simulink model "testifintegratoriscorrect"  (R2019a)
settings: Solver=FixedStepAuto  StartTime=0.0  StopTime=100  FixedStep=1e-4  RelTol=1e-5
InitFcn:
  | HeightAboveSeaLevel = 400 * rand;
  | Temperature = 288.15 + 30 * (rand - 0.5);
  | Pressure = 	101325 + 6000 * (rand - 0.5);
  | 
  | GustStart = 5 * rand;
  | GustLength = [100 + 50 * (rand - 0.5), 100 + 50 * (rand - 0.5), 100 + 50 * (rand - 0.5)];
  | GuestAmplitude = [ 10 * (rand - 0.5), 10 * (rand - 0.5),  10 * (rand - 0.5)];
  | 
  | ShearSpeed = 20 * rand;
  | ShearDirection = 360 * rand;
  | 
  | HeightAboveSeaLevel = 5.4419142084;
  | Temperature = 288.15;
  | Pressure = 	101325;
  | 
  | GustStart = 2.5;
  | GustLength = [100, 100, 100];
  | GuestAmplitude = [ 2.5, -2.5,  1];
  | 
  | ShearSpeed = 10;
  | ShearDirection = 180;
values from neighbouring files (symbols this model uses):
  D = zeros(size(B))    [RocketOutputFunction.m]    (also in StateSpaceController.m = zeros(13, 3); TimeDelayCompensationElevator.m = [0; 0])
  F = eye(6)    [MEKFAttitudeOnly.m]
  Ki2 = lqr(Ai2, Bi2, Q, R)    [StateSpaceController.m]
  q = x(13:16)    [AdaptiveLQR.m]    (also in MEKF.m = nominal_state(4:7); MEKFAttitudeOnly.m = [1 0 0 0]; MEKF_old.m = nominal_state(4:7); NonlinearStateEstimationForActuatorDelay.m = x(4:7))
  r = sym('r', [3 1])    [StateSpaceController.m]    (also in TimeDelayCompensationElevator.m = [0;0]; Tracker.m = [0; 0; -(rocket_length - Average_cg)])
  s = linspace(0, 100, nums)    [ImpactVelocityFunction.m]    (also in ImpactVelocityNotParallelMatlab.m = 1:5:500; ParallelImpactVelocity.m = .1:.01:500; ParralelRun.m = linspace(5,7, nums); RunImpactVelocityParforCompiled.m = 1:0.1:500)
undefined symbols (not defined in the file or in its folder): deg, e0_0, e1_0, e2_0, e3_0, Earth, Light, magnitude, MIL, rad, WGS84
libraries: aerolibutil x10, simulink x9, aerolibconvert2 x7, sharedtransform x7, shared6dof x7, aerolibwind2 x3, sharedutil x3, aerolibfltsims x2, aerolibasang x2, shared6dofsys x2, aerolibatmos2 x1, aerolibbdyn x1
(part 2 of 2)

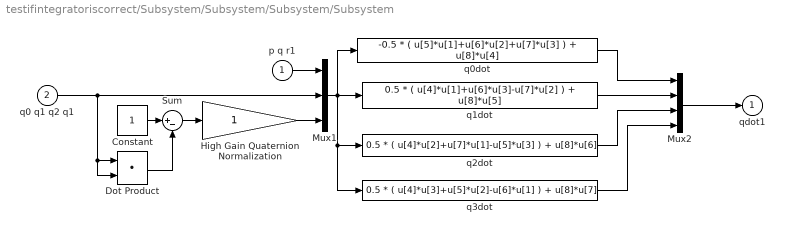
== system testifintegratoriscorrect/Subsystem/Subsystem/Subsystem/Subsystem ==
  p q r1 : Inport
  q0 q1 q2 q1 : Inport  Port=2
  Constant : Constant
  Dot Product : DotProduct  OutDataTypeStr=Inherit: Inherit via internal rule
  High Gain Quaternion Normalization : Gain  SaturateOnIntegerOverflow=on  OutDataTypeStr=Inherit: Same as input  ParamDataTypeStr=Inherit: Same as input
  Mux1 : Mux  Inputs=[3 4 1]
  Mux2 : Mux
  Sum : Sum  Inputs=|+-  SaturateOnIntegerOverflow=on  InputSameDT=on  OutDataTypeStr=Inherit: Same as first input
  q0dot : Fcn  Expr=-0.5 * ( u[5]*u[1]+u[6]*u[2]+u[7]*u[3] ) + u[8]*u[4]
  q1dot : Fcn  Expr=0.5 * ( u[4]*u[1]+u[6]*u[3]-u[7]*u[2] ) + u[8]*u[5]
  q2dot : Fcn  Expr=0.5 * ( u[4]*u[2]+u[7]*u[1]-u[5]*u[3] ) + u[8]*u[6]
  q3dot : Fcn  Expr=0.5 * ( u[4]*u[3]+u[5]*u[2]-u[6]*u[1] ) + u[8]*u[7]
  qdot1 : Outport  InitialOutput=0
  wires:
  Constant/1 -> Sum/1
  Dot Product/1 -> Sum/2
  Mux1/1 -> q2dot/1, q3dot/1, q0dot/1, q1dot/1
  q0 q1 q2 q1/1 -> Dot Product/1, Dot Product/2, Mux1/2
  Sum/1 -> High Gain Quaternion Normalization/1
  Mux2/1 -> qdot1/1
  q0dot/1 -> Mux2/1
  q3dot/1 -> Mux2/4
  q1dot/1 -> Mux2/2
  q2dot/1 -> Mux2/3
  High Gain Quaternion Normalization/1 -> Mux1/3
  p q r1/1 -> Mux1/1

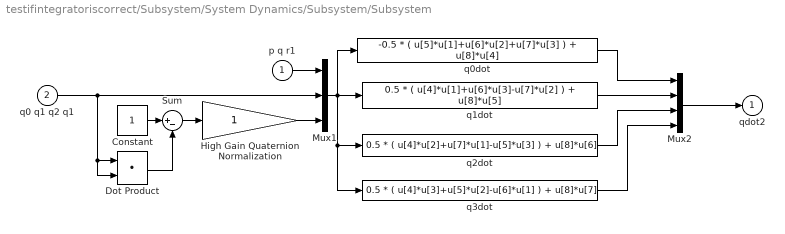
== system testifintegratoriscorrect/Subsystem/System Dynamics/Subsystem/Subsystem ==
  p q r1 : Inport
  q0 q1 q2 q1 : Inport  Port=2
  Constant : Constant
  Dot Product : DotProduct  OutDataTypeStr=Inherit: Inherit via internal rule
  High Gain Quaternion Normalization : Gain  SaturateOnIntegerOverflow=on  OutDataTypeStr=Inherit: Same as input  ParamDataTypeStr=Inherit: Same as input
  Mux1 : Mux  Inputs=[3 4 1]
  Mux2 : Mux
  Sum : Sum  Inputs=|+-  SaturateOnIntegerOverflow=on  InputSameDT=on  OutDataTypeStr=Inherit: Same as first input
  q0dot : Fcn  Expr=-0.5 * ( u[5]*u[1]+u[6]*u[2]+u[7]*u[3] ) + u[8]*u[4]
  q1dot : Fcn  Expr=0.5 * ( u[4]*u[1]+u[6]*u[3]-u[7]*u[2] ) + u[8]*u[5]
  q2dot : Fcn  Expr=0.5 * ( u[4]*u[2]+u[7]*u[1]-u[5]*u[3] ) + u[8]*u[6]
  q3dot : Fcn  Expr=0.5 * ( u[4]*u[3]+u[5]*u[2]-u[6]*u[1] ) + u[8]*u[7]
  qdot2 : Outport
  wires:
  q0 q1 q2 q1/1 -> Dot Product/1, Dot Product/2, Mux1/2
  Mux1/1 -> q2dot/1, q3dot/1, q0dot/1, q1dot/1
  Constant/1 -> Sum/1
  High Gain Quaternion Normalization/1 -> Mux1/3
  q1dot/1 -> Mux2/2
  q0dot/1 -> Mux2/1
  Sum/1 -> High Gain Quaternion Normalization/1
  Dot Product/1 -> Sum/2
  q3dot/1 -> Mux2/4
  Mux2/1 -> qdot2/1
  q2dot/1 -> Mux2/3
  p q r1/1 -> Mux1/1

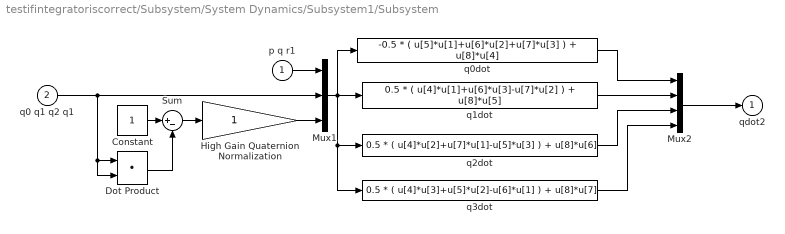
== system testifintegratoriscorrect/Subsystem/System Dynamics/Subsystem1/Subsystem ==
  p q r1 : Inport
  q0 q1 q2 q1 : Inport  Port=2
  Constant : Constant
  Dot Product : DotProduct  OutDataTypeStr=Inherit: Inherit via internal rule
  High Gain Quaternion Normalization : Gain  SaturateOnIntegerOverflow=on  OutDataTypeStr=Inherit: Same as input  ParamDataTypeStr=Inherit: Same as input
  Mux1 : Mux  Inputs=[3 4 1]
  Mux2 : Mux
  Sum : Sum  Inputs=|+-  SaturateOnIntegerOverflow=on  InputSameDT=on  OutDataTypeStr=Inherit: Same as first input
  q0dot : Fcn  Expr=-0.5 * ( u[5]*u[1]+u[6]*u[2]+u[7]*u[3] ) + u[8]*u[4]
  q1dot : Fcn  Expr=0.5 * ( u[4]*u[1]+u[6]*u[3]-u[7]*u[2] ) + u[8]*u[5]
  q2dot : Fcn  Expr=0.5 * ( u[4]*u[2]+u[7]*u[1]-u[5]*u[3] ) + u[8]*u[6]
  q3dot : Fcn  Expr=0.5 * ( u[4]*u[3]+u[5]*u[2]-u[6]*u[1] ) + u[8]*u[7]
  qdot2 : Outport
  wires:
  q0 q1 q2 q1/1 -> Dot Product/1, Dot Product/2, Mux1/2
  Mux1/1 -> q2dot/1, q3dot/1, q0dot/1, q1dot/1
  Constant/1 -> Sum/1
  High Gain Quaternion Normalization/1 -> Mux1/3
  q1dot/1 -> Mux2/2
  q0dot/1 -> Mux2/1
  Sum/1 -> High Gain Quaternion Normalization/1
  Dot Product/1 -> Sum/2
  q3dot/1 -> Mux2/4
  Mux2/1 -> qdot2/1
  q2dot/1 -> Mux2/3
  p q r1/1 -> Mux1/1

== matlab function testifintegratoriscorrect/50Hz delay ==
  settings: updateMethod=DISCRETE
  data: time input; input input; delayed_input output
function delayed_input = Servo(time, input)
    persistent lastupdate
    if isempty(lastupdate)
        lastupdate = [0;0];
    end
    
    servo_frequency = 50; %Hz
    if mod(time, 1/servo_frequency) == 0
        lastupdate = input;
    end    
        
    delayed_input = lastupdate;
end

== matlab function testifintegratoriscorrect/Subsystem/Acceleration Calculator/Subsystem/AngleOfAtack1 ==
  settings: updateMethod=DISCRETE
  data: Airspeed input; AoA output
function AoA = AngleOfAttack(Airspeed)
    AoA = acos(Airspeed(3) / norm(Airspeed));
        
    if norm(Airspeed) <= .01
        AoA = 0;
    end
end

== matlab function testifintegratoriscorrect/Subsystem/Acceleration Calculator/Forces And Moments simple model1 ==
  settings: updateMethod=DISCRETE
  data: Mach input; Airspeed input size=[3 1]; AoA input; Density input; Temperature input; DynamicPressure input; CenterOfMassX input; Thrust input; Forces output; body_angular_velocity input; Xe input; Moments output
function [Forces, Moments]  = forces(Mach, Airspeed, AoA, Density, Temperature, DynamicPressure, CenterOfMassX, Thrust, body_angular_velocity, Xe)
    persistent ThetaRotation
    if isempty(ThetaRotation)
         ThetaRotation = eye(3);
    end
    
    %% Rocket Shape Constants
    Reference_Diameter = 7.62e-2;
    Reference_Radius = Reference_Diameter / 2;
    Reference_Area = Reference_Radius^2 * pi;
    
    NoseCone_Length = 15e-2;
    BodyTube_Length = 80e-2; 
    NoseCone_WetArea = pi * Reference_Radius * NoseCone_Length;          % pi*r*l 
    BodyTube_WetArea = pi * Reference_Radius * 2 * BodyTube_Length;      % pi*d*l
    NoseCone_PlanformArea = Reference_Diameter * NoseCone_Length / 2;
    BodyTube_PlanformArea = Reference_Diameter * BodyTube_Length;
    
    SurfaceRoughness = 20e-6;
    
    sinphi = Reference_Radius / hypot(Reference_Radius, NoseCone_Length);
    BodyTube_CP = 0.55;
    NoseCone_CP = 0.1;
    PitchCenterX = 0;
   
    
    COT_to_COM = .95 - CenterOfMassX; %get actual value and change over time as solid motor burns
    
    %% General Constants
    K = 1.1;
   
    %% Coefficients
    angularrate_local = ThetaRotation \ body_angular_velocity;
    [CN, Cpitch] = CalculatePitchAndNormalCDs(Mach, K, Reference_Diameter, AoA, Airspeed, angularrate_local(2), NoseCone_Length, BodyTube_Length, Reference_Area, CenterOfMassX, PitchCenterX, NoseCone_PlanformArea, BodyTube_PlanformArea, NoseCone_CP, BodyTube_CP);

    Cbase = .12 + .13*Mach^2;
    CFrictionDrag = CalculateFrictionDrag(Temperature, Density, Reference_Radius, Reference_Area, SurfaceRoughness, NoseCone_Length, BodyTube_Length, Airspeed, Mach, NoseCone_WetArea, BodyTube_WetArea);
    Cpressure = PressureDragForce(sinphi);
    
    Cdrag = Cbase + CFrictionDrag + Cpressure;
    Caxial = AxialDragMul(AoA) * Cdrag;

    Cyaw = 0;
    %Croll = 0.003 * (rand - 0.5);
    Croll = 0;
    Cside = 0;
    
     %% Random Noise to pitch and yaw coefficients in the range of +- 5e-4
    %Cpitch = Cpitch + .1 * (rand - 0.5);
    %Cyaw = Cyaw + .1 * (rand - 0.5);
    %Croll = Croll + .00005 * (rand - 0.5);
    %% Forces and Moments
    lengtha = norm(Airspeed(1:2));
    
    sina = Airspeed(2) / lengtha;
    cosa = Airspeed(1) / lengtha;

    ThetaRotation = [cosa, -sina, 0; sina, cosa, 0; 0, 0, 1];
    
    z = DynamicPressure * Reference_Area;
    Thrust_moment = COT_to_COM * [Thrust(2); Thrust(1); 0];
    
    Forces = ThetaRotation * z * -[CN; Cside; Caxial] + Thrust;
    Moments = ThetaRotation * (z * Reference_Diameter * [-Cyaw; Cpitch; Croll]) + Thrust_moment;
    
    if Xe(3) <= 0
        Forces = [0;0;Forces(3)];
        Moments = [0; 0; 0];
    end
    
end

== matlab function testifintegratoriscorrect/Subsystem2/Desired Quaternion ==
  settings: updateMethod=DISCRETE
  data: input_acceleration input; thrust_acceleration input; desired_quaternion output size=[1 4]; ln_quat output
function [desired_quaternion, ln_quat] = func(input_acceleration, thrust_acceleration)

    max_horizontal_acceleration = sin(deg2rad(10)) * thrust_acceleration;
    if norm(input_acceleration) > max_horizontal_acceleration
        input_acceleration = input_acceleration * max_horizontal_acceleration / norm(input_acceleration);
    end
    
    global_thrust = [input_acceleration.', (thrust_acceleration^2 - norm(input_acceleration)^2)^.5];
    
    if norm(global_thrust) == 0
        global_thrust = [0,0,1];
    end
    
    desired_quaternion = quatnormalize([ global_thrust(3) + norm(global_thrust), cross([0;0;1], global_thrust) ]);
%     test = quatnormalize([norm(global_thrust) + global_thrust(3), cross([0 0 1], global_thrust)]);
    
    if norm(desired_quaternion(2:4)) == 0
        ln_quat = [0 0 0];
    else
        ln_quat = desired_quaternion(2:4)/norm(desired_quaternion(2:4)) * desired_quaternion(1);
    end
    
%     desired_quaternion = [cos(pi/8) sin(pi/8) * [1 0 0]];

== matlab function testifintegratoriscorrect/Desired Quaternion ==
  settings: updateMethod=DISCRETE
  data: current_orientation input; desired_quaternion input; current_quaternion output size=[1 4]
function current_quaternion = func(current_orientation, desired_quaternion)
    rotation_b = quatmultiply(quatinv(current_orientation.'), desired_quaternion); %rotation required in body coordinate system

    theta = atan( rotation_b(4) / rotation_b(1) ); %half the roll angle
    roll_b = [cos(theta), 0, 0, sin(theta)]; %extract roll part of quaternion
    noroll_b = quatmultiply(rotation_b, quatinv(roll_b)); %desired rotation in body coordinate system
%     noroll_i = quatmultiply(current_orientation.', quatmultiply(noroll_b, quatinv(current_orientation.')));
    
    current_quaternion = quatnormalize(quatinv( noroll_b )); % then take the inverse to pretend to be at inverse orientation, due to state space being designed like that

    if current_quaternion(1) < 0
        current_quaternion = -current_quaternion;
    end

== matlab function testifintegratoriscorrect/Subsystem/System Dynamics/w to quat ==
  settings: updateMethod=DISCRETE
  data: w input; quaternion output size=[1 4]
function quaternion = func(w)
    quaternion = [cos(norm(w) / 2), sin(norm(w) / 2) * w.' / norm(w)];

== matlab function testifintegratoriscorrect/Subsystem/Desired Quaternion ==
  settings: updateMethod=DISCRETE
  data: current_orientation input; current_quaternion output
function current_quaternion = func(current_orientation)
    current_quaternion = current_orientation;
    
    t = acos(current_quaternion(1));
    if current_quaternion(1) < 0
        current_quaternion(1) = cos(pi - t);
        current_quaternion(2:4) = -current_quaternion(2:4);
    end

== matlab function testifintegratoriscorrect/Subsystem/Acceleration Calculator/Subsystem/Subsystem/DCM ==
  settings: updateMethod=DISCRETE
  data: DCM output
function DCM  = forces
    DCM = [1,0,0;0,1,0;0,0,1];

== matlab function testifintegratoriscorrect/Subsystem/Acceleration Calculator/Subsystem/Subsystem/MATLAB Function ==
  data: u input; magnitude output
function magnitude = VectorNorm(u)
    magnitude = norm(u);
